simulink model "task_2_model"  (R2021a)
settings: Solver=VariableStepAuto  StartTime=0.0  StopTime=50.0  RelTol=1e-3
values from neighbouring files (symbols this model uses):
  d_1 = 0.01    [task_2_parameters.m]
  d_2 = 0.01    [task_2_parameters.m]
  g = 0.666666666667    [C.mat]    (also in task_2_parameters.m = 9.82)
  L = 1    [C.mat]    (also in task_2_parameters.m)
  m_c = 1.5    [task_2_parameters.m]
  m_p = 0.5    [task_2_parameters.m]
settings Model: Creator=vedan  LastModifiedBy=vedan

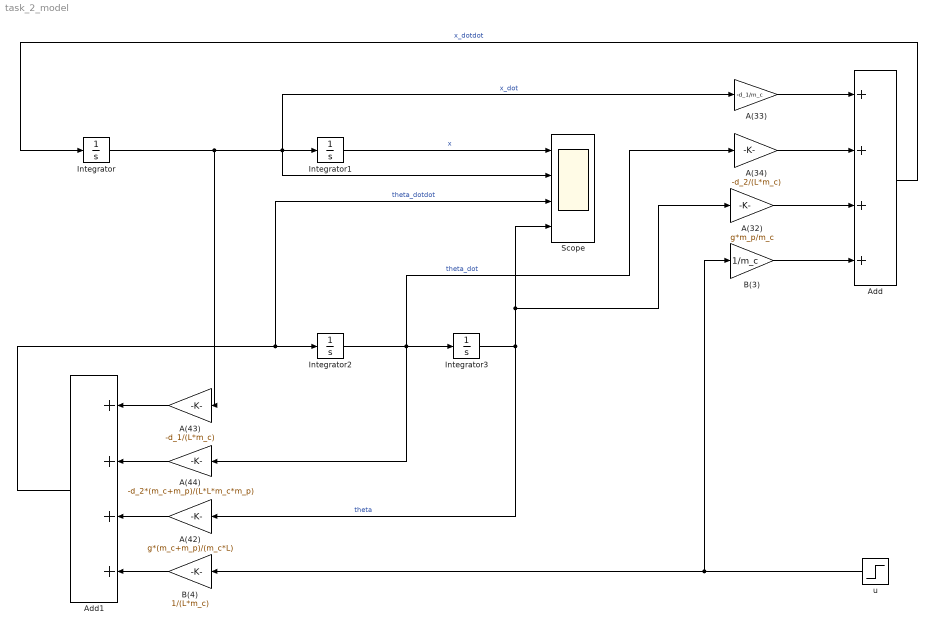
== system task_2_model ==
  A(32) : Gain  Gain=g*m_p/m_c
  A(33) : Gain  Gain=-d_1/m_c
  A(34) : Gain  Gain=-d_2/(L*m_c)
  A(42) : Gain  Gain=g*(m_c+m_p)/(m_c*L)
  A(43) : Gain  Gain=-d_1/(L*m_c)
  A(44) : Gain  Gain=-d_2*(m_c+m_p)/(L*L*m_c*m_p)
  Add : Sum  Inputs=++++
  Add1 : Sum  Inputs=++++
  B(3) : Gain  Gain=1/m_c
  B(4) : Gain  Gain=1/(L*m_c)
  Integrator{,1..3} (4 alike) : Integrator
  Scope : Scope  NumInputPorts=4
  u : Step  SampleTime=0
  wires:
  Integrator/1 -> A(43)/1, Scope/2, A(33)/1, Integrator1/1  "x_dot"
  Integrator2/1 -> A(44)/1, A(34)/1, Integrator3/1  "theta_dot"
  Add/1 -> Integrator/1  "x_dotdot"
  Add1/1 -> Scope/3, Integrator2/1  "theta_dotdot"
  Integrator3/1 -> A(32)/1, Scope/4, A(42)/1  "theta"
  Integrator1/1 -> Scope/1  "x"
  A(33)/1 -> Add/1
  A(34)/1 -> Add/2
  B(3)/1 -> Add/4
  A(32)/1 -> Add/3
  u/1 -> B(3)/1, B(4)/1
  A(43)/1 -> Add1/1
  A(44)/1 -> Add1/2
  A(42)/1 -> Add1/3
  B(4)/1 -> Add1/4
